simulink model "lab9punk1"  (R2022b)
settings: Solver=VariableStepAuto  StartTime=0.0  StopTime=10.0  RelTol=1e-3
settings Model: Creator=Wikor  LastModifiedBy=mateu
settings DebuggingCC: UnconnectedInputMsg=warning  UnconnectedOutputMsg=warning  UnconnectedLineMsg=warning
settings ModelReferenceCC: EnableRefExpFcnMdlSchedulingChecks=on
settings RTWCC: DLArmComputeVersion=19.05

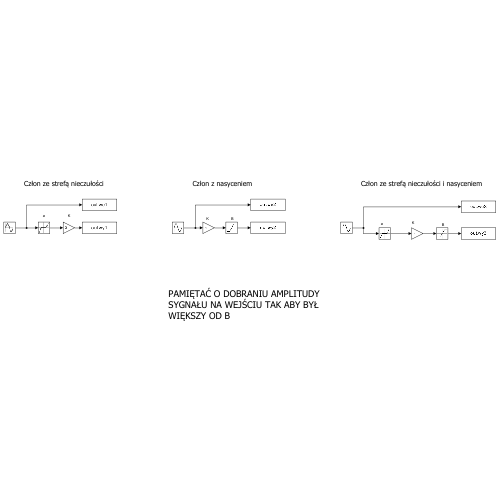
[thumbnail: Simulink's stored preview of the top-level diagram]
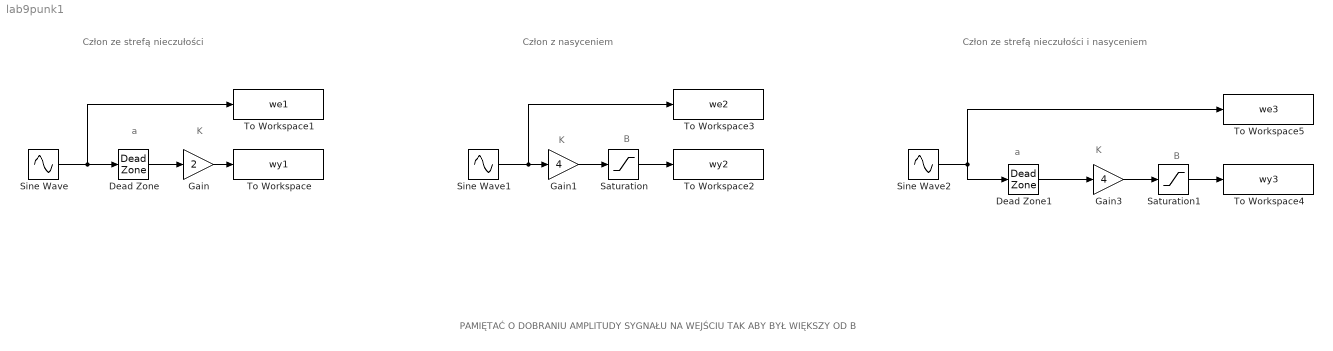
== system lab9punk1 ==
  note: B
  note: K
  note: a
  note: K
  note: a
  note: PAMIĘTAĆ O DOBRANIU AMPLITUDY SYGNAŁU NA WEJŚCIU TAK ABY BYŁ WIĘKSZY OD B
  note: B
  note: K
  note: Człon ze strefą nieczułości
  note: Człon z nasyceniem
  note: Człon ze strefą nieczułości i nasyceniem
  Dead Zone : DeadZone  LowerValue=-2.8  UpperValue=2.8
  Dead Zone1 : DeadZone  LowerValue=-1.5  UpperValue=1.5
  Gain : Gain  Gain=2
  Gain1 : Gain  Gain=4
  Gain3 : Gain  Gain=4
  Saturation : Saturate  UpperLimit=5  LowerLimit=-5
  Saturation1 : Saturate  UpperLimit=4  LowerLimit=-4
  Sine Wave : Sin  Amplitude=6  SampleTime=0
  Sine Wave1 : Sin  Amplitude=11  SampleTime=0
  Sine Wave2 : Sin  Amplitude=5  SampleTime=0
  To Workspace : ToWorkspace  VariableName=wy1  SampleTime=-1
  To Workspace1 : ToWorkspace  VariableName=we1  SampleTime=-1
  To Workspace2 : ToWorkspace  VariableName=wy2  SampleTime=-1
  To Workspace3 : ToWorkspace  VariableName=we2  SampleTime=-1
  To Workspace4 : ToWorkspace  VariableName=wy3  SampleTime=-1
  To Workspace5 : ToWorkspace  VariableName=we3  SampleTime=-1
  wires:
  Sine Wave/1 -> To Workspace1/1, Dead Zone/1
  Dead Zone/1 -> Gain/1
  Gain/1 -> To Workspace/1
  Sine Wave1/1 -> Gain1/1, To Workspace3/1
  Sine Wave2/1 -> To Workspace5/1, Dead Zone1/1
  Gain1/1 -> Saturation/1
  Saturation/1 -> To Workspace2/1
  Dead Zone1/1 -> Gain3/1
  Gain3/1 -> Saturation1/1
  Saturation1/1 -> To Workspace4/1
